simulink model "Drone2_simulink"  (R2024a)
settings: Solver=ode1be  StartTime=0.0  StopTime=1000  FixedStep=0.001  MaxStep=0.001  MinStep=0.00095  RelTol=1e-3
PreLoadFcn:
  | Drone_data;
model workspace: external: MATLAB File C:\Users\admin\OneDrive - Indian Institute of Technology Jodhpur\IIT JODHPUR\Research Work\Amphibious Drone\MATLAB_CODE\2025\New_Drone\Drone_1\Drone1_simulink_DataFile.m (data not in the file)
undefined symbols (not defined in the file): Environment, Newton, Raphson, Vehicle, X, Y, Z
libraries: sm_lib x1684, nesl_utility x63, slpidlib x25, eeGeneralControl x6, matrix_library x3, rllib x2, simulink x2, fl_lib x1, sharedutil x1, SignalEditorBlockLib x1
(part 3 of 17)

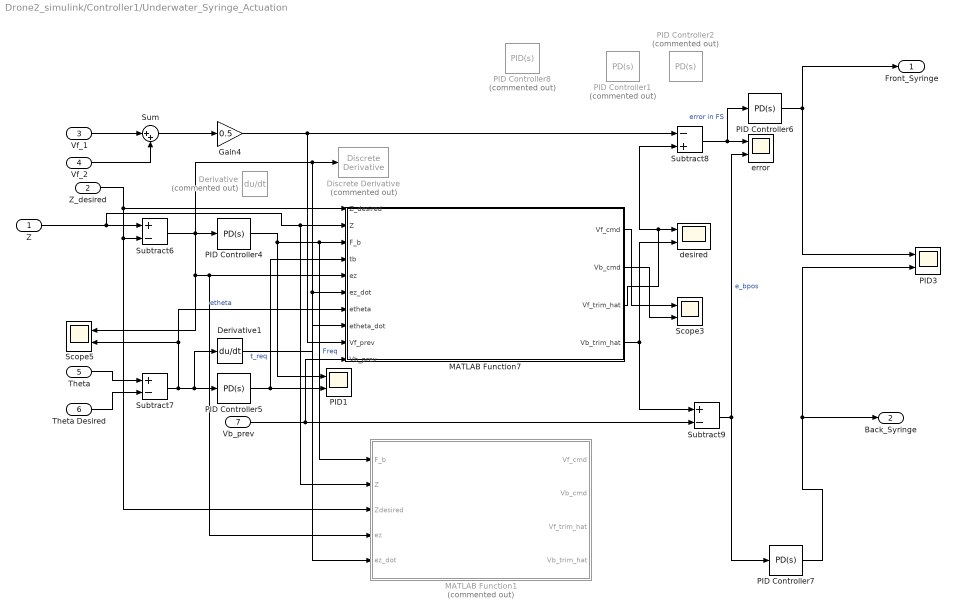
== system Drone2_simulink/Controller1/Underwater_Syringe_Actuation ==
  Z : Inport
  Z_desired : Inport  Port=2
  Vf_1 : Inport  Port=3
  Vf_2 : Inport  Port=4
  Theta : Inport  Port=5
  Theta Desired : Inport  Port=6
  Vb_prev : Inport  Port=7
  Derivative : Derivative  Commented=on
  Derivative1 : Derivative
  Discrete Derivative : simulink/Discrete/Discrete Derivative  Commented=on  gainval=1.0  ICPrevScaledInput=0.0  OutMin=[]  OutMax=[]  OutDataType=fixdt(1, 16)  OutScaling=2^-10  DoSatur=off
  Gain4 : Gain  Gain=0.5
  MATLAB Function1 : MATLAB Function  Commented=on  TreatAsAtomicUnit=on  mask{V_MIN=Vehicle.Syringe.Front.minpos, V_MAX=Vehicle.Syringe.Front.maxpos, V_DOT_MAX=0.012, HF=0.2, A=0, g=9.81, rho=1000, dt=0.001, Kp_pos=0.002, Kp_vel=0.002, Kr=0.005, EZDB=0.05, sigma=0.1, Ez_high=1, PLRate=0.0002, PKRate=0.05, ETDB=3}
      mask prompts: V_MIN "Min"; V_MAX "Max"; V_DOT_MAX "max rate"; HF "Half Length of drone"; A "Area of Syringe"; g "Gravity"; rho "Density"; dt "Sample Time"; Kp_pos "Learning Rate-Pose"; Kp_vel "Slow Learning Rate"; Kr "K_Rate"; EZDB "Error zone to reduce adaption"; sigma "Steady state error region"; Ez_high "mode switch region"; PLRate "Pitch Learning Rate"; PKRate "K_Rate"; ETDB "Error zone to reduce adaption"
  MATLAB Function7 : MATLAB Function  TreatAsAtomicUnit=on  mask{Min=Vehicle.Syringe.Front.minpos, Max=Vehicle.Syringe.Front.maxpos, HF=0.2, AS=0, G=9.81, RHO=1000, DT=0.001, DFRate=0.02, DMRate=0.002, DSRate=0.002, Dpanelty=0.005, EZDB=0.05, PLRate=0.0002, PKRate=0.05, ETDB=3}
      mask prompts: HF "Half Length of drone"; AS "Area of Syringe"; G "Gravity"; RHO "Density"; DT "Sample Time"; DFRate "Fast Learning rate with |e|>1"; DMRate "Medium Learning Rate"; DSRate "Slow Learning Rate"; Dpanelty "K_Rate"; EZDB "Error zone to reduce adaption"; PLRate "Pitch Learning Rate"; PKRate "K_Rate"; ETDB "Error zone to reduce adaption"
  PID Controller1 : slpidlib/PID Controller  Commented=on  Controller=PD  Form=Parallel  TimeDomain=Continuous-time  UseExternalTs=off  SampleTime=-1  IntegratorMethod=Forward Euler  FilterMethod=Forward Euler  ControllerParametersSource=internal  P=3500.0200194669353  I=843.52365195509  UseKiTs=on  D=26.9299392102605  UseExternalDerivativeSource=off  N=0.579906738639273  UseFilter=on  TunerSelectOption=Transfer Function Based (PID Tuner App)  InitialConditionSource=internal  InitialConditionForIntegrator=0  InitialConditionForFilter=0  DifferentiatorICPrevScaledInput=0  ExternalReset=none  TrackingMode=off  Kt=1  LimitOutput=on  SatLimitsSource=internal  UpperSaturationLimit=40  LowerSaturationLimit=0  LinearizeAsGain=on  AntiWindupMode=none  Kb=1  LimitIntegrator=off  UpperIntegratorSaturationLimit=inf  LowerIntegratorSaturationLimit=-inf  POutMin=[]  POutMax=[]  IOutMin=[]  IOutMax=[]  DOutMin=[]  DOutMax=[]  NOutMin=[]  NOutMax=[]  SumOutMin=[]  SumOutMax=[]  SaturationOutMin=[]  SaturationOutMax=[]  PParamMin=[]  PParamMax=[]  IParamMin=[]  IParamMax=[]  DParamMin=[]  DParamMax=[]  NParamMin=[]  NParamMax=[]  KbParamMin=[]  KbParamMax=[]  KtParamMin=[]  KtParamMax=[]  KbOutMin=[]  KbOutMax=[]  KtOutMin=[]  KtOutMax=[]  IntegratorOutMin=[]  IntegratorOutMax=[]  FilterOutMin=[]  FilterOutMax=[]  SumI1OutMin=[]  SumI1OutMax=[]  SumI2OutMin=[]  SumI2OutMax=[]  SumI3OutMin=[]  SumI3OutMax=[]  SumI4OutMin=[]  SumI4OutMax=[]  SumDOutMin=[]  SumDOutMax=[]  DifferentiatorOutMin=[]  DifferentiatorOutMax=[]  FilterDiffOutCoefMin=[]  FilterDiffOutCoefMax=[]  ReciprocalOutMin=[]  ReciprocalOutMax=[]  SumDenOutMin=[]  SumDenOutMax=[]  SumNumOutMin=[]  SumNumOutMax=[]  DivideOutMin=[]  DivideOutMax=[]  UdiffTsProdOutMin=[]  UdiffTsProdOutMax=[]  NTsProdOutMin=[]  NTsProdOutMax=[]  UintegralTsProdOutMin=[]  UintegralTsProdOutMax=[]  UngainTsProdOutMin=[]  UngainTsProdOutMax=[]  ClampingZeroOutDataTypeStr=Inherit: Inherit via back propagation  ClampingZeroOutMin=[]  ClampingZeroOutMax=[]  FilterDenConstantOutDataTypeStr=Inherit: Inherit via back propagation  FilterDenConstantOutMin=[]  FilterDenConstantOutMax=[]  PCopyOutDataTypeStr=Inherit: Inherit via back propagation  PCopyOutMin=[]  PCopyOutMax=[]  NCopyOutDataTypeStr=Inherit: Inherit via back propagation  NCopyOutMin=[]  NCopyOutMax=[]  IntegratorContinuousStateAttributes=''  IntegratorStateMustResolveToSignalObject=off  IntegratorRTWStateStorageClass=Auto  FilterContinuousStateAttributes=''  FilterStateMustResolveToSignalObject=off  FilterRTWStateStorageClass=Auto  ParallelPVariant=InternalParameters  IdealPVariant=Disabled  IVariant=Disabled  DVariant=InternalParameters  IntegratorVariant=Disabled  SatVariant=Enabled  AWVariant=Disabled  PCopyVariant=Disabled  TRVariant=Disabled  FdbkBlocksVariant=Forward  IdealPFdbkVariant=Disabled  SatFdbkVariant=Disabled  DerivativeFilterVariant=ContFilter  NVariant=InternalParameters  NCopyVariant=Disabled  FilterICVariant=InternalICsFilter  IntegratorICVariant=Disabled  ExternalResetVariant=Disabled  TRSumVariant=Passthrough  SumFdbkVariant=Disabled  SumVariant=Sum_PD  TsampFilterVariant=InternalTs  TsampNgainVariant=Passthrough  TsampIntegralVariant=Disabled_SignalSpec  ExternalSaturationOutDataTypeStr=Inherit: Same as second input  DerivativeSourceVariant=ErrorSignal
  PID Controller2 : slpidlib/PID Controller  Commented=on  Controller=PD  Form=Parallel  TimeDomain=Continuous-time  UseExternalTs=off  SampleTime=-1  IntegratorMethod=Forward Euler  FilterMethod=Forward Euler  ControllerParametersSource=internal  P=3744.13110896654  I=964.677966952311  UseKiTs=on  D=30  UseExternalDerivativeSource=off  N=0.58  UseFilter=on  TunerSelectOption=Transfer Function Based (PID Tuner App)  InitialConditionSource=internal  InitialConditionForIntegrator=0  InitialConditionForFilter=0  DifferentiatorICPrevScaledInput=0  ExternalReset=none  TrackingMode=off  Kt=1  LimitOutput=on  SatLimitsSource=internal  UpperSaturationLimit=40  LowerSaturationLimit=0  LinearizeAsGain=on  AntiWindupMode=none  Kb=1  LimitIntegrator=off  UpperIntegratorSaturationLimit=inf  LowerIntegratorSaturationLimit=-inf  POutMin=[]  POutMax=[]  IOutMin=[]  IOutMax=[]  DOutMin=[]  DOutMax=[]  NOutMin=[]  NOutMax=[]  SumOutMin=[]  SumOutMax=[]  SaturationOutMin=[]  SaturationOutMax=[]  PParamMin=[]  PParamMax=[]  IParamMin=[]  IParamMax=[]  DParamMin=[]  DParamMax=[]  NParamMin=[]  NParamMax=[]  KbParamMin=[]  KbParamMax=[]  KtParamMin=[]  KtParamMax=[]  KbOutMin=[]  KbOutMax=[]  KtOutMin=[]  KtOutMax=[]  IntegratorOutMin=[]  IntegratorOutMax=[]  FilterOutMin=[]  FilterOutMax=[]  SumI1OutMin=[]  SumI1OutMax=[]  SumI2OutMin=[]  SumI2OutMax=[]  SumI3OutMin=[]  SumI3OutMax=[]  SumI4OutMin=[]  SumI4OutMax=[]  SumDOutMin=[]  SumDOutMax=[]  DifferentiatorOutMin=[]  DifferentiatorOutMax=[]  FilterDiffOutCoefMin=[]  FilterDiffOutCoefMax=[]  ReciprocalOutMin=[]  ReciprocalOutMax=[]  SumDenOutMin=[]  SumDenOutMax=[]  SumNumOutMin=[]  SumNumOutMax=[]  DivideOutMin=[]  DivideOutMax=[]  UdiffTsProdOutMin=[]  UdiffTsProdOutMax=[]  NTsProdOutMin=[]  NTsProdOutMax=[]  UintegralTsProdOutMin=[]  UintegralTsProdOutMax=[]  UngainTsProdOutMin=[]  UngainTsProdOutMax=[]  ClampingZeroOutDataTypeStr=Inherit: Inherit via back propagation  ClampingZeroOutMin=[]  ClampingZeroOutMax=[]  FilterDenConstantOutDataTypeStr=Inherit: Inherit via back propagation  FilterDenConstantOutMin=[]  FilterDenConstantOutMax=[]  PCopyOutDataTypeStr=Inherit: Inherit via back propagation  PCopyOutMin=[]  PCopyOutMax=[]  NCopyOutDataTypeStr=Inherit: Inherit via back propagation  NCopyOutMin=[]  NCopyOutMax=[]  IntegratorContinuousStateAttributes=''  IntegratorStateMustResolveToSignalObject=off  IntegratorRTWStateStorageClass=Auto  FilterContinuousStateAttributes=''  FilterStateMustResolveToSignalObject=off  FilterRTWStateStorageClass=Auto  ParallelPVariant=InternalParameters  IdealPVariant=Disabled  IVariant=Disabled  DVariant=InternalParameters  IntegratorVariant=Disabled  SatVariant=Enabled  AWVariant=Disabled  PCopyVariant=Disabled  TRVariant=Disabled  FdbkBlocksVariant=Forward  IdealPFdbkVariant=Disabled  SatFdbkVariant=Disabled  DerivativeFilterVariant=ContFilter  NVariant=InternalParameters  NCopyVariant=Disabled  FilterICVariant=InternalICsFilter  IntegratorICVariant=Disabled  ExternalResetVariant=Disabled  TRSumVariant=Passthrough  SumFdbkVariant=Disabled  SumVariant=Sum_PD  TsampFilterVariant=InternalTs  TsampNgainVariant=Passthrough  TsampIntegralVariant=Disabled_SignalSpec  ExternalSaturationOutDataTypeStr=Inherit: Same as second input  DerivativeSourceVariant=ErrorSignal
  PID Controller4 : slpidlib/PID Controller  Controller=PD  Form=Parallel  TimeDomain=Continuous-time  UseExternalTs=off  SampleTime=-1  IntegratorMethod=Forward Euler  FilterMethod=Forward Euler  ControllerParametersSource=internal  P=8  I=0  UseKiTs=on  D=0.5  UseExternalDerivativeSource=off  N=20  UseFilter=on  TunerSelectOption=Transfer Function Based (PID Tuner App)  InitialConditionSource=internal  InitialConditionForIntegrator=0  InitialConditionForFilter=0  DifferentiatorICPrevScaledInput=0  ExternalReset=none  TrackingMode=off  Kt=1  LimitOutput=off  SatLimitsSource=internal  UpperSaturationLimit=Vehicle.Syringe.Thrustlim  LowerSaturationLimit=-Vehicle.Syringe.Thrustlim  LinearizeAsGain=on  AntiWindupMode=none  Kb=1  LimitIntegrator=off  UpperIntegratorSaturationLimit=inf  LowerIntegratorSaturationLimit=-inf  POutMin=[]  POutMax=[]  IOutMin=[]  IOutMax=[]  DOutMin=[]  DOutMax=[]  NOutMin=[]  NOutMax=[]  SumOutMin=[]  SumOutMax=[]  SaturationOutMin=[]  SaturationOutMax=[]  PParamMin=[]  PParamMax=[]  IParamMin=[]  IParamMax=[]  DParamMin=[]  DParamMax=[]  NParamMin=[]  NParamMax=[]  KbParamMin=[]  KbParamMax=[]  KtParamMin=[]  KtParamMax=[]  KbOutMin=[]  KbOutMax=[]  KtOutMin=[]  KtOutMax=[]  IntegratorOutMin=[]  IntegratorOutMax=[]  FilterOutMin=[]  FilterOutMax=[]  SumI1OutMin=[]  SumI1OutMax=[]  SumI2OutMin=[]  SumI2OutMax=[]  SumI3OutMin=[]  SumI3OutMax=[]  SumI4OutMin=[]  SumI4OutMax=[]  SumDOutMin=[]  SumDOutMax=[]  DifferentiatorOutMin=[]  DifferentiatorOutMax=[]  FilterDiffOutCoefMin=[]  FilterDiffOutCoefMax=[]  ReciprocalOutMin=[]  ReciprocalOutMax=[]  SumDenOutMin=[]  SumDenOutMax=[]  SumNumOutMin=[]  SumNumOutMax=[]  DivideOutMin=[]  DivideOutMax=[]  UdiffTsProdOutMin=[]  UdiffTsProdOutMax=[]  NTsProdOutMin=[]  NTsProdOutMax=[]  UintegralTsProdOutMin=[]  UintegralTsProdOutMax=[]  UngainTsProdOutMin=[]  UngainTsProdOutMax=[]  ClampingZeroOutDataTypeStr=Inherit: Inherit via back propagation  ClampingZeroOutMin=[]  ClampingZeroOutMax=[]  FilterDenConstantOutDataTypeStr=Inherit: Inherit via back propagation  FilterDenConstantOutMin=[]  FilterDenConstantOutMax=[]  PCopyOutDataTypeStr=Inherit: Inherit via back propagation  PCopyOutMin=[]  PCopyOutMax=[]  NCopyOutDataTypeStr=Inherit: Inherit via back propagation  NCopyOutMin=[]  NCopyOutMax=[]  IntegratorContinuousStateAttributes=''  IntegratorStateMustResolveToSignalObject=off  IntegratorRTWStateStorageClass=Auto  FilterContinuousStateAttributes=''  FilterStateMustResolveToSignalObject=off  FilterRTWStateStorageClass=Auto  ParallelPVariant=InternalParameters  IdealPVariant=Disabled  IVariant=Disabled  DVariant=InternalParameters  IntegratorVariant=Disabled  SatVariant=Disabled  AWVariant=Disabled  PCopyVariant=Disabled  TRVariant=Disabled  FdbkBlocksVariant=Forward  IdealPFdbkVariant=Disabled  SatFdbkVariant=Disabled  DerivativeFilterVariant=ContFilter  NVariant=InternalParameters  NCopyVariant=Disabled  FilterICVariant=InternalICsFilter  IntegratorICVariant=Disabled  ExternalResetVariant=Disabled  TRSumVariant=Passthrough  SumFdbkVariant=Disabled  SumVariant=Sum_PD  TsampFilterVariant=InternalTs  TsampNgainVariant=Passthrough  TsampIntegralVariant=Disabled_SignalSpec  ExternalSaturationOutDataTypeStr=Inherit: Same as second input  DerivativeSourceVariant=ErrorSignal
  PID Controller5 : slpidlib/PID Controller  Controller=PD  Form=Parallel  TimeDomain=Continuous-time  UseExternalTs=off  SampleTime=-1  IntegratorMethod=Forward Euler  FilterMethod=Forward Euler  ControllerParametersSource=internal  P=4  I=0  UseKiTs=on  D=0.5  UseExternalDerivativeSource=off  N=100  UseFilter=on  TunerSelectOption=Transfer Function Based (PID Tuner App)  InitialConditionSource=internal  InitialConditionForIntegrator=0  InitialConditionForFilter=0  DifferentiatorICPrevScaledInput=0  ExternalReset=none  TrackingMode=off  Kt=1  LimitOutput=off  SatLimitsSource=internal  UpperSaturationLimit=Vehicle.Syringe.Thrustlim  LowerSaturationLimit=-Vehicle.Syringe.Thrustlim  LinearizeAsGain=on  AntiWindupMode=none  Kb=1  LimitIntegrator=off  UpperIntegratorSaturationLimit=inf  LowerIntegratorSaturationLimit=-inf  POutMin=[]  POutMax=[]  IOutMin=[]  IOutMax=[]  DOutMin=[]  DOutMax=[]  NOutMin=[]  NOutMax=[]  SumOutMin=[]  SumOutMax=[]  SaturationOutMin=[]  SaturationOutMax=[]  PParamMin=[]  PParamMax=[]  IParamMin=[]  IParamMax=[]  DParamMin=[]  DParamMax=[]  NParamMin=[]  NParamMax=[]  KbParamMin=[]  KbParamMax=[]  KtParamMin=[]  KtParamMax=[]  KbOutMin=[]  KbOutMax=[]  KtOutMin=[]  KtOutMax=[]  IntegratorOutMin=[]  IntegratorOutMax=[]  FilterOutMin=[]  FilterOutMax=[]  SumI1OutMin=[]  SumI1OutMax=[]  SumI2OutMin=[]  SumI2OutMax=[]  SumI3OutMin=[]  SumI3OutMax=[]  SumI4OutMin=[]  SumI4OutMax=[]  SumDOutMin=[]  SumDOutMax=[]  DifferentiatorOutMin=[]  DifferentiatorOutMax=[]  FilterDiffOutCoefMin=[]  FilterDiffOutCoefMax=[]  ReciprocalOutMin=[]  ReciprocalOutMax=[]  SumDenOutMin=[]  SumDenOutMax=[]  SumNumOutMin=[]  SumNumOutMax=[]  DivideOutMin=[]  DivideOutMax=[]  UdiffTsProdOutMin=[]  UdiffTsProdOutMax=[]  NTsProdOutMin=[]  NTsProdOutMax=[]  UintegralTsProdOutMin=[]  UintegralTsProdOutMax=[]  UngainTsProdOutMin=[]  UngainTsProdOutMax=[]  ClampingZeroOutDataTypeStr=Inherit: Inherit via back propagation  ClampingZeroOutMin=[]  ClampingZeroOutMax=[]  FilterDenConstantOutDataTypeStr=Inherit: Inherit via back propagation  FilterDenConstantOutMin=[]  FilterDenConstantOutMax=[]  PCopyOutDataTypeStr=Inherit: Inherit via back propagation  PCopyOutMin=[]  PCopyOutMax=[]  NCopyOutDataTypeStr=Inherit: Inherit via back propagation  NCopyOutMin=[]  NCopyOutMax=[]  IntegratorContinuousStateAttributes=''  IntegratorStateMustResolveToSignalObject=off  IntegratorRTWStateStorageClass=Auto  FilterContinuousStateAttributes=''  FilterStateMustResolveToSignalObject=off  FilterRTWStateStorageClass=Auto  ParallelPVariant=InternalParameters  IdealPVariant=Disabled  IVariant=Disabled  DVariant=InternalParameters  IntegratorVariant=Disabled  SatVariant=Disabled  AWVariant=Disabled  PCopyVariant=Disabled  TRVariant=Disabled  FdbkBlocksVariant=Forward  IdealPFdbkVariant=Disabled  SatFdbkVariant=Disabled  DerivativeFilterVariant=ContFilter  NVariant=InternalParameters  NCopyVariant=Disabled  FilterICVariant=InternalICsFilter  IntegratorICVariant=Disabled  ExternalResetVariant=Disabled  TRSumVariant=Passthrough  SumFdbkVariant=Disabled  SumVariant=Sum_PD  TsampFilterVariant=InternalTs  TsampNgainVariant=Passthrough  TsampIntegralVariant=Disabled_SignalSpec  ExternalSaturationOutDataTypeStr=Inherit: Same as second input  DerivativeSourceVariant=ErrorSignal
  PID Controller6 : slpidlib/PID Controller  Controller=PD  Form=Parallel  TimeDomain=Continuous-time  UseExternalTs=off  SampleTime=-1  IntegratorMethod=Forward Euler  FilterMethod=Forward Euler  ControllerParametersSource=internal  P=3500  I=843.52365195509  UseKiTs=on  D=30  UseExternalDerivativeSource=off  N=1  UseFilter=on  TunerSelectOption=Transfer Function Based (PID Tuner App)  InitialConditionSource=internal  InitialConditionForIntegrator=0  InitialConditionForFilter=0  DifferentiatorICPrevScaledInput=0  ExternalReset=none  TrackingMode=off  Kt=1  LimitOutput=on  SatLimitsSource=internal  UpperSaturationLimit=40  LowerSaturationLimit=0  LinearizeAsGain=on  AntiWindupMode=none  Kb=1  LimitIntegrator=off  UpperIntegratorSaturationLimit=inf  LowerIntegratorSaturationLimit=-inf  POutMin=[]  POutMax=[]  IOutMin=[]  IOutMax=[]  DOutMin=[]  DOutMax=[]  NOutMin=[]  NOutMax=[]  SumOutMin=[]  SumOutMax=[]  SaturationOutMin=[]  SaturationOutMax=[]  PParamMin=[]  PParamMax=[]  IParamMin=[]  IParamMax=[]  DParamMin=[]  DParamMax=[]  NParamMin=[]  NParamMax=[]  KbParamMin=[]  KbParamMax=[]  KtParamMin=[]  KtParamMax=[]  KbOutMin=[]  KbOutMax=[]  KtOutMin=[]  KtOutMax=[]  IntegratorOutMin=[]  IntegratorOutMax=[]  FilterOutMin=[]  FilterOutMax=[]  SumI1OutMin=[]  SumI1OutMax=[]  SumI2OutMin=[]  SumI2OutMax=[]  SumI3OutMin=[]  SumI3OutMax=[]  SumI4OutMin=[]  SumI4OutMax=[]  SumDOutMin=[]  SumDOutMax=[]  DifferentiatorOutMin=[]  DifferentiatorOutMax=[]  FilterDiffOutCoefMin=[]  FilterDiffOutCoefMax=[]  ReciprocalOutMin=[]  ReciprocalOutMax=[]  SumDenOutMin=[]  SumDenOutMax=[]  SumNumOutMin=[]  SumNumOutMax=[]  DivideOutMin=[]  DivideOutMax=[]  UdiffTsProdOutMin=[]  UdiffTsProdOutMax=[]  NTsProdOutMin=[]  NTsProdOutMax=[]  UintegralTsProdOutMin=[]  UintegralTsProdOutMax=[]  UngainTsProdOutMin=[]  UngainTsProdOutMax=[]  ClampingZeroOutDataTypeStr=Inherit: Inherit via back propagation  ClampingZeroOutMin=[]  ClampingZeroOutMax=[]  FilterDenConstantOutDataTypeStr=Inherit: Inherit via back propagation  FilterDenConstantOutMin=[]  FilterDenConstantOutMax=[]  PCopyOutDataTypeStr=Inherit: Inherit via back propagation  PCopyOutMin=[]  PCopyOutMax=[]  NCopyOutDataTypeStr=Inherit: Inherit via back propagation  NCopyOutMin=[]  NCopyOutMax=[]  IntegratorContinuousStateAttributes=''  IntegratorStateMustResolveToSignalObject=off  IntegratorRTWStateStorageClass=Auto  FilterContinuousStateAttributes=''  FilterStateMustResolveToSignalObject=off  FilterRTWStateStorageClass=Auto  ParallelPVariant=InternalParameters  IdealPVariant=Disabled  IVariant=Disabled  DVariant=InternalParameters  IntegratorVariant=Disabled  SatVariant=Enabled  AWVariant=Disabled  PCopyVariant=Disabled  TRVariant=Disabled  FdbkBlocksVariant=Forward  IdealPFdbkVariant=Disabled  SatFdbkVariant=Disabled  DerivativeFilterVariant=ContFilter  NVariant=InternalParameters  NCopyVariant=Disabled  FilterICVariant=InternalICsFilter  IntegratorICVariant=Disabled  ExternalResetVariant=Disabled  TRSumVariant=Passthrough  SumFdbkVariant=Disabled  SumVariant=Sum_PD  TsampFilterVariant=InternalTs  TsampNgainVariant=Passthrough  TsampIntegralVariant=Disabled_SignalSpec  ExternalSaturationOutDataTypeStr=Inherit: Same as second input  DerivativeSourceVariant=ErrorSignal
  PID Controller7 : slpidlib/PID Controller  Controller=PD  Form=Parallel  TimeDomain=Continuous-time  UseExternalTs=off  SampleTime=-1  IntegratorMethod=Forward Euler  FilterMethod=Forward Euler  ControllerParametersSource=internal  P=3750  I=964.677966952311  UseKiTs=on  D=30  UseExternalDerivativeSource=off  N=1  UseFilter=on  TunerSelectOption=Transfer Function Based (PID Tuner App)  InitialConditionSource=internal  InitialConditionForIntegrator=0  InitialConditionForFilter=0  DifferentiatorICPrevScaledInput=0  ExternalReset=none  TrackingMode=off  Kt=1  LimitOutput=on  SatLimitsSource=internal  UpperSaturationLimit=40  LowerSaturationLimit=0  LinearizeAsGain=on  AntiWindupMode=none  Kb=1  LimitIntegrator=off  UpperIntegratorSaturationLimit=inf  LowerIntegratorSaturationLimit=-inf  POutMin=[]  POutMax=[]  IOutMin=[]  IOutMax=[]  DOutMin=[]  DOutMax=[]  NOutMin=[]  NOutMax=[]  SumOutMin=[]  SumOutMax=[]  SaturationOutMin=[]  SaturationOutMax=[]  PParamMin=[]  PParamMax=[]  IParamMin=[]  IParamMax=[]  DParamMin=[]  DParamMax=[]  NParamMin=[]  NParamMax=[]  KbParamMin=[]  KbParamMax=[]  KtParamMin=[]  KtParamMax=[]  KbOutMin=[]  KbOutMax=[]  KtOutMin=[]  KtOutMax=[]  IntegratorOutMin=[]  IntegratorOutMax=[]  FilterOutMin=[]  FilterOutMax=[]  SumI1OutMin=[]  SumI1OutMax=[]  SumI2OutMin=[]  SumI2OutMax=[]  SumI3OutMin=[]  SumI3OutMax=[]  SumI4OutMin=[]  SumI4OutMax=[]  SumDOutMin=[]  SumDOutMax=[]  DifferentiatorOutMin=[]  DifferentiatorOutMax=[]  FilterDiffOutCoefMin=[]  FilterDiffOutCoefMax=[]  ReciprocalOutMin=[]  ReciprocalOutMax=[]  SumDenOutMin=[]  SumDenOutMax=[]  SumNumOutMin=[]  SumNumOutMax=[]  DivideOutMin=[]  DivideOutMax=[]  UdiffTsProdOutMin=[]  UdiffTsProdOutMax=[]  NTsProdOutMin=[]  NTsProdOutMax=[]  UintegralTsProdOutMin=[]  UintegralTsProdOutMax=[]  UngainTsProdOutMin=[]  UngainTsProdOutMax=[]  ClampingZeroOutDataTypeStr=Inherit: Inherit via back propagation  ClampingZeroOutMin=[]  ClampingZeroOutMax=[]  FilterDenConstantOutDataTypeStr=Inherit: Inherit via back propagation  FilterDenConstantOutMin=[]  FilterDenConstantOutMax=[]  PCopyOutDataTypeStr=Inherit: Inherit via back propagation  PCopyOutMin=[]  PCopyOutMax=[]  NCopyOutDataTypeStr=Inherit: Inherit via back propagation  NCopyOutMin=[]  NCopyOutMax=[]  IntegratorContinuousStateAttributes=''  IntegratorStateMustResolveToSignalObject=off  IntegratorRTWStateStorageClass=Auto  FilterContinuousStateAttributes=''  FilterStateMustResolveToSignalObject=off  FilterRTWStateStorageClass=Auto  ParallelPVariant=InternalParameters  IdealPVariant=Disabled  IVariant=Disabled  DVariant=InternalParameters  IntegratorVariant=Disabled  SatVariant=Enabled  AWVariant=Disabled  PCopyVariant=Disabled  TRVariant=Disabled  FdbkBlocksVariant=Forward  IdealPFdbkVariant=Disabled  SatFdbkVariant=Disabled  DerivativeFilterVariant=ContFilter  NVariant=InternalParameters  NCopyVariant=Disabled  FilterICVariant=InternalICsFilter  IntegratorICVariant=Disabled  ExternalResetVariant=Disabled  TRSumVariant=Passthrough  SumFdbkVariant=Disabled  SumVariant=Sum_PD  TsampFilterVariant=InternalTs  TsampNgainVariant=Passthrough  TsampIntegralVariant=Disabled_SignalSpec  ExternalSaturationOutDataTypeStr=Inherit: Same as second input  DerivativeSourceVariant=ErrorSignal
  PID Controller8 : slpidlib/PID Controller  Commented=on  Controller=PID  Form=Parallel  TimeDomain=Continuous-time  UseExternalTs=off  SampleTime=-1  IntegratorMethod=Forward Euler  FilterMethod=Forward Euler  ControllerParametersSource=internal  P=44.1440048797783  I=843.52365195509  UseKiTs=on  D=0  UseExternalDerivativeSource=off  N=100  UseFilter=on  TunerSelectOption=Transfer Function Based (PID Tuner App)  InitialConditionSource=internal  InitialConditionForIntegrator=0  InitialConditionForFilter=0  DifferentiatorICPrevScaledInput=0  ExternalReset=none  TrackingMode=off  Kt=1  LimitOutput=on  SatLimitsSource=internal  UpperSaturationLimit=40  LowerSaturationLimit=0  LinearizeAsGain=on  AntiWindupMode=none  Kb=1  LimitIntegrator=off  UpperIntegratorSaturationLimit=inf  LowerIntegratorSaturationLimit=-inf  POutMin=[]  POutMax=[]  IOutMin=[]  IOutMax=[]  DOutMin=[]  DOutMax=[]  NOutMin=[]  NOutMax=[]  SumOutMin=[]  SumOutMax=[]  SaturationOutMin=[]  SaturationOutMax=[]  PParamMin=[]  PParamMax=[]  IParamMin=[]  IParamMax=[]  DParamMin=[]  DParamMax=[]  NParamMin=[]  NParamMax=[]  KbParamMin=[]  KbParamMax=[]  KtParamMin=[]  KtParamMax=[]  KbOutMin=[]  KbOutMax=[]  KtOutMin=[]  KtOutMax=[]  IntegratorOutMin=[]  IntegratorOutMax=[]  FilterOutMin=[]  FilterOutMax=[]  SumI1OutMin=[]  SumI1OutMax=[]  SumI2OutMin=[]  SumI2OutMax=[]  SumI3OutMin=[]  SumI3OutMax=[]  SumI4OutMin=[]  SumI4OutMax=[]  SumDOutMin=[]  SumDOutMax=[]  DifferentiatorOutMin=[]  DifferentiatorOutMax=[]  FilterDiffOutCoefMin=[]  FilterDiffOutCoefMax=[]  ReciprocalOutMin=[]  ReciprocalOutMax=[]  SumDenOutMin=[]  SumDenOutMax=[]  SumNumOutMin=[]  SumNumOutMax=[]  DivideOutMin=[]  DivideOutMax=[]  UdiffTsProdOutMin=[]  UdiffTsProdOutMax=[]  NTsProdOutMin=[]  NTsProdOutMax=[]  UintegralTsProdOutMin=[]  UintegralTsProdOutMax=[]  UngainTsProdOutMin=[]  UngainTsProdOutMax=[]  ClampingZeroOutDataTypeStr=Inherit: Inherit via back propagation  ClampingZeroOutMin=[]  ClampingZeroOutMax=[]  FilterDenConstantOutDataTypeStr=Inherit: Inherit via back propagation  FilterDenConstantOutMin=[]  FilterDenConstantOutMax=[]  PCopyOutDataTypeStr=Inherit: Inherit via back propagation  PCopyOutMin=[]  PCopyOutMax=[]  NCopyOutDataTypeStr=Inherit: Inherit via back propagation  NCopyOutMin=[]  NCopyOutMax=[]  IntegratorContinuousStateAttributes=''  IntegratorStateMustResolveToSignalObject=off  IntegratorRTWStateStorageClass=Auto  FilterContinuousStateAttributes=''  FilterStateMustResolveToSignalObject=off  FilterRTWStateStorageClass=Auto  ParallelPVariant=InternalParameters  IdealPVariant=Disabled  IVariant=InternalParameters  DVariant=InternalParameters  IntegratorVariant=Continuous  SatVariant=Enabled  AWVariant=Passthrough  PCopyVariant=Disabled  TRVariant=Disabled  FdbkBlocksVariant=Forward  IdealPFdbkVariant=Disabled  SatFdbkVariant=Disabled  DerivativeFilterVariant=ContFilter  NVariant=InternalParameters  NCopyVariant=Disabled  FilterICVariant=InternalICsFilter  IntegratorICVariant=InternalICs  ExternalResetVariant=Disabled  TRSumVariant=Passthrough  SumFdbkVariant=Disabled  SumVariant=Sum_PID  TsampFilterVariant=InternalTs  TsampNgainVariant=Passthrough  TsampIntegralVariant=Disabled_SignalSpec  ExternalSaturationOutDataTypeStr=Inherit: Same as second input  DerivativeSourceVariant=ErrorSignal
  PID1 : Scope  NumInputPorts=2
  PID3 : Scope  NumInputPorts=2
  Scope3 : Scope  NumInputPorts=2
  Scope5 : Scope  NumInputPorts=2
  Subtract6 : Sum  Inputs=+-
  Subtract7 : Sum  Inputs=+-
  Subtract8 : Sum  Inputs=-+
  Subtract9 : Sum  Inputs=+-
  Sum : Sum  Inputs=|++
  desired : Scope  NumInputPorts=2
  error : Scope  NumInputPorts=2
  Front_Syringe : Outport
  Back_Syringe : Outport  Port=2
  wires:
  Subtract6/1 -> PID Controller4/1, MATLAB Function7/5(ez), MATLAB Function1/4(ez), Scope5/1, MATLAB Function7/6(ez_dot), MATLAB Function1/5(ez_dot), Discrete Derivative/1
  Z_desired/1 -> Subtract6/2, MATLAB Function1/3(Zdesired), MATLAB Function7/1(Z_desired)
  PID Controller7/1 -> Back_Syringe/1, PID3/2
  PID Controller6/1 -> Front_Syringe/1, PID3/1
  MATLAB Function7/4(Vb_trim_hat) -> desired/2, Subtract9/1
  MATLAB Function7/3(Vf_trim_hat) -> desired/1, Subtract8/2
  Vb_prev/1 -> MATLAB Function7/10(Vb_prev), Subtract9/2
  PID Controller5/1 -> PID1/2, MATLAB Function7/4(tb)  "t_req"
  MATLAB Function7/1(Vf_cmd) -> Scope3/1
  Derivative1/1 -> MATLAB Function7/8(etheta_dot)
  PID Controller4/1 -> PID1/1, MATLAB Function7/3(F_b), MATLAB Function1/1(F_b)  "Freq"
  Gain4/1 -> MATLAB Function7/9(Vf_prev), Subtract8/1
  Subtract7/1 -> PID Controller5/1, Derivative1/1, MATLAB Function7/7(etheta), Scope5/2  "etheta"
  Theta Desired/1 -> Subtract7/2
  Theta/1 -> Subtract7/1
  Sum/1 -> Gain4/1
  Z/1 -> Subtract6/1, MATLAB Function7/2(Z), MATLAB Function1/2(Z)
  Subtract8/1 -> PID Controller6/1, error/1  "error in FS"
  MATLAB Function7/2(Vb_cmd) -> Scope3/2
  Vf_2/1 -> Sum/2
  Vf_1/1 -> Sum/1
  Subtract9/1 -> PID Controller7/1, error/2  "e_bpos"

== system Drone2_simulink/Drive Controls/Thrust Controls ==
  Bus Element In : Inport  PortName=Reference  Element=Speed
  Bus Element In2 : Inport  PortName=Reference  Element=Depth
  Bus Element In7 : Inport  PortName=Reference  Element=Heading
  Bus Element In1 : Inport  Port=2  PortName=VehicleFDBK  Element=COM.Body.Vb.u
  Bus Element In8 : Inport  Port=2  PortName=VehicleFDBK  Element=COM.Body.Vb.v
  Bus Element In5 : Inport  Port=2  PortName=VehicleFDBK  Element=COM.Body.wb
  Bus Element In6 : Inport  Port=2  PortName=VehicleFDBK  Element=COM.Derived.Euler
  Bus Element In3 : Inport  Port=2  PortName=VehicleFDBK  Element=COM.Derived.Euler.theta
  Bus Element In4 : Inport  Port=2  PortName=VehicleFDBK  Element=COM.World.Xe.Z
  Depth and Pitch Control : Subsystem
  Heading and Yaw Control : Subsystem
  Longitudinal Speed (Surge) Control : Subsystem
  PPf : Outport
  SPf : Outport  Port=2
  BVTf : Outport  Port=3
  SVTf : Outport  Port=4
  BHTf : Outport  Port=5
  SHTf : Outport  Port=6
  wires:
  Longitudinal Speed (Surge) Control/1(PPfcmd) -> Depth and Pitch Control/1(PPf), PPf/1
  Bus Element In/1 -> Longitudinal Speed (Surge) Control/1(uRef)
  Bus Element In1/1 -> Longitudinal Speed (Surge) Control/2(u)
  Longitudinal Speed (Surge) Control/2(SPfcmd) -> Depth and Pitch Control/2(SPf), SPf/1
  Depth and Pitch Control/2(SVTfcmd) -> SVTf/1
  Depth and Pitch Control/1(BVTfcmd) -> BVTf/1
  Heading and Yaw Control/1(BHTfcmd) -> BHTf/1
  Heading and Yaw Control/2(SHTfcmd) -> SHTf/1
  Bus Element In2/1 -> Depth and Pitch Control/3(ZRef)
  Bus Element In3/1 -> Depth and Pitch Control/5(theta)
  Bus Element In4/1 -> Depth and Pitch Control/4(Z)
  Bus Element In5/1 -> Heading and Yaw Control/3(pqr)
  Bus Element In6/1 -> Heading and Yaw Control/4(phithetapsi)
  Bus Element In7/1 -> Heading and Yaw Control/2(psiRef)
  Bus Element In8/1 -> Heading and Yaw Control/1(v)

== system Drone2_simulink/Drive Controls/Torque Controls ==
  Tbht (N*m) : Constant  Value=0
  Tbvt (N*m) : Constant  Value=0
  Tpp (N*m) : Constant  Value=0
  Tsht (N*m) : Constant  Value=0
  Tsp (N*m) : Constant  Value=0
  Tsvt (N*m) : Constant  Value=0
  BHTt : Outport
  BVTt : Outport  Port=2
  PPt : Outport  Port=3
  SPt : Outport  Port=4
  SHTt : Outport  Port=5
  SVTt : Outport  Port=6
  wires:
  Tbht (N*m)/1 -> BHTt/1
  Tsvt (N*m)/1 -> SVTt/1
  Tpp (N*m)/1 -> PPt/1
  Tsp (N*m)/1 -> SPt/1
  Tbvt (N*m)/1 -> BVTt/1
  Tsht (N*m)/1 -> SHTt/1

== system Drone2_simulink/Hydrostatic & Hydrodynamic Effects/Added Mass Forces ==
  Vb : Inport
  wb : Inport  Port=2
  Abb : Inport  Port=3
  dwbdt : Inport  Port=4
  Added Mass : Subsystem
  Added Mass Matrix : Constant  Value=Vehicle.AddedMassMatrix
  Coriolis : Subsystem
  Scope : Scope  NumInputPorts=2
  Scope1 : Scope  NumInputPorts=2
  Bus Element Out : Outport  PortName=AddedMass  Element=AMForcesXYZ
  Bus Element Out1 : Outport  PortName=AddedMass  Element=AMMomentsXYZ
  Bus Element Out2 : Outport  PortName=AddedMass  Element=CForcesXYZ
  Bus Element Out3 : Outport  PortName=AddedMass  Element=CMomentsXYZ
  wires:
  Added Mass Matrix/1 -> Added Mass/1(Ma), Coriolis/3(Ma)
  Abb/1 -> Added Mass/2(Abb)
  dwbdt/1 -> Added Mass/3(dwbdt)
  Added Mass/1(Fxyz) -> Scope/2, Bus Element Out/1
  Added Mass/2(Mxyz) -> Scope1/2, Bus Element Out1/1
  Vb/1 -> Coriolis/1(Vb)
  wb/1 -> Coriolis/2(wb)
  Coriolis/2(Mxyz) -> Scope1/1, Bus Element Out3/1
  Coriolis/1(Fxyz) -> Scope/1, Bus Element Out2/1

== system Drone2_simulink/Hydrostatic & Hydrodynamic Effects/Buoyancy Force ==
  Z : Inport
  Constant : Constant  Value=-Vehicle.Dist.CGtoTop
  Constant1 : Constant  Value=Vehicle.Dist.CGtoBottom
  Constant2 : Constant
  Constant3 : Constant  Value=0
  Constant4 : Constant  Value=Vehicle.MaxBuoyancyForce
  MATLAB Function : MATLAB Function  TreatAsAtomicUnit=on
  Product : Product
  Saturation : Saturate  UpperLimit=Vehicle.Dist.CGtoBottom  LowerLimit=-Vehicle.Dist.CGtoTop
  Scope : Scope  NumInputPorts=2
  Buoyancy force : Outport
  wires:
  Constant/1 -> MATLAB Function/2(a)
  Constant3/1 -> MATLAB Function/6(reverse), MATLAB Function/5(y_b)
  Constant4/1 -> Product/2
  Z/1 -> Saturation/1
  Constant1/1 -> MATLAB Function/3(b)
  Constant2/1 -> MATLAB Function/4(y_a)
  MATLAB Function/1(Factor) -> Product/1, Scope/1
  Product/1 -> Scope/2, Buoyancy force/1
  Saturation/1 -> MATLAB Function/1(Z)

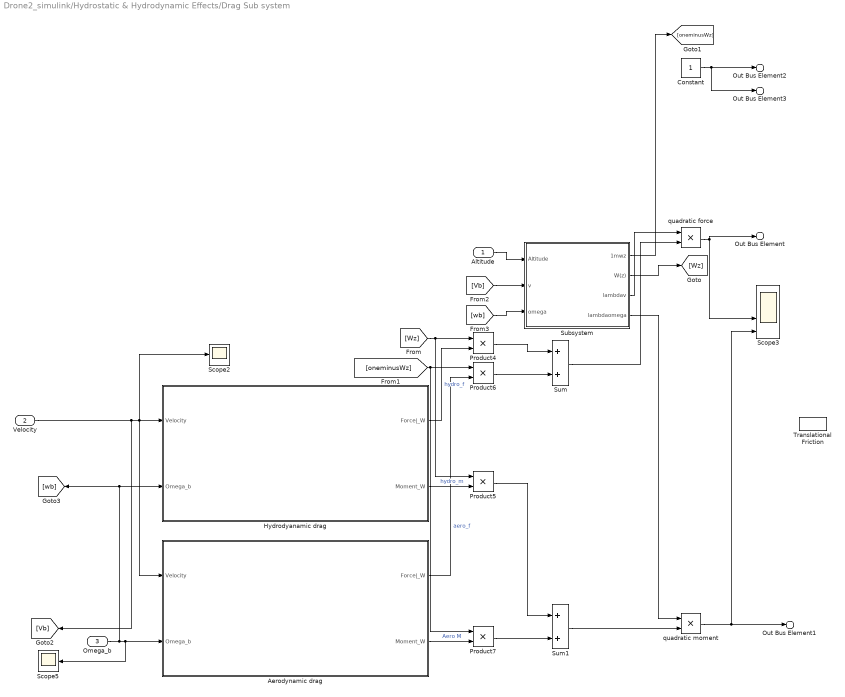
== system Drone2_simulink/Hydrostatic & Hydrodynamic Effects/Drag Sub system ==
  Altitude : Inport
  Velocity : Inport  Port=2
  Omega_b : Inport  Port=3
  Aerodynamic drag : Subsystem
  Constant : Constant
  Hydrodyanamic drag : Subsystem
  Product{4..7} (4 alike) : Product
  Scope2 : Scope
  Scope3 : Scope  NumInputPorts=4
  Scope5 : Scope
  Subsystem : Subsystem
  Sum : Sum
  Sum1 : Sum
  Translational Friction : fl_lib/Mechanical/Translational Elements/Translational Friction  brkwy_frc=25 N  brkwy_vel=0.1 m/s  Col_frc=20 N  visc_coef=100 N*s/m  v_specify=off  v_priority=None  v=0 m/s  v_nominal_specify=off  v_nominal_value=1  v_nominal_unit=m/s  f_specify=off  f_priority=None  f=0 N  f_nominal_specify=off  f_nominal_value=1  f_nominal_unit=N
      settings: InternalSimscapePortConfiguration="{\"Bottom\":[],\"Left\":[{\"id\":\"R\",\"label\":\"R\",\"type\":\"foundation.mechanical.translational.translational\"}],\"Right\":[{\"id\":\"C\",\"label\":\"C\",\"type\":\"foundation.mechanical.translational.translational\"}],\"Top\":[]}"
  quadratic force : Product
  quadratic moment : Product
  Out Bus Element : Outport  PortName=Drag  Element=Forces
  Out Bus Element1 : Outport  PortName=Drag  Element=Moments
  Out Bus Element2 : Outport  PortName=Drag  Element=LinearForce
  Out Bus Element3 : Outport  PortName=Drag  Element=LinearMoment
  wires:
  [oneminusWz] -> Product6/1, Product7/1
  Omega_b/1 -> Aerodynamic drag/2(Omega_b), Scope5/1, Hydrodyanamic drag/2(Omega_b), [wb]
  Velocity/1 -> Scope2/1, Hydrodyanamic drag/1(Velocity), Aerodynamic drag/1(Velocity), [Vb]
  Sum/1 -> quadratic force/2
  [Wz] -> Product4/1, Product5/1
  Hydrodyanamic drag/1(Force|_W) -> Product4/2  "hydro_f"
  quadratic force/1 -> Out Bus Element/1, Scope3/3
  Hydrodyanamic drag/2(Moment_W) -> Product5/2  "hydro_m"
  Aerodynamic drag/1(Force|_W) -> Product6/2  "aero_f"
  Aerodynamic drag/2(Moment_W) -> Product7/2  "Aero M"
  Subsystem/4(lambdaomega) -> quadratic moment/1
  Product6/1 -> Sum/2
  Altitude/1 -> Subsystem/1(Altitude)
  Product7/1 -> Sum1/2
  [Vb] -> Subsystem/2(v)
  Sum1/1 -> quadratic moment/2
  Product5/1 -> Sum1/1
  [wb] -> Subsystem/3(omega)
  Product4/1 -> Sum/1
  Subsystem/1(1mwz) -> [oneminusWz]
  Subsystem/2(W(z)) -> [Wz]
  Subsystem/3(lambdav) -> quadratic force/1
  quadratic moment/1 -> Out Bus Element1/1, Scope3/4
  Constant/1 -> Out Bus Element3/1, Out Bus Element2/1

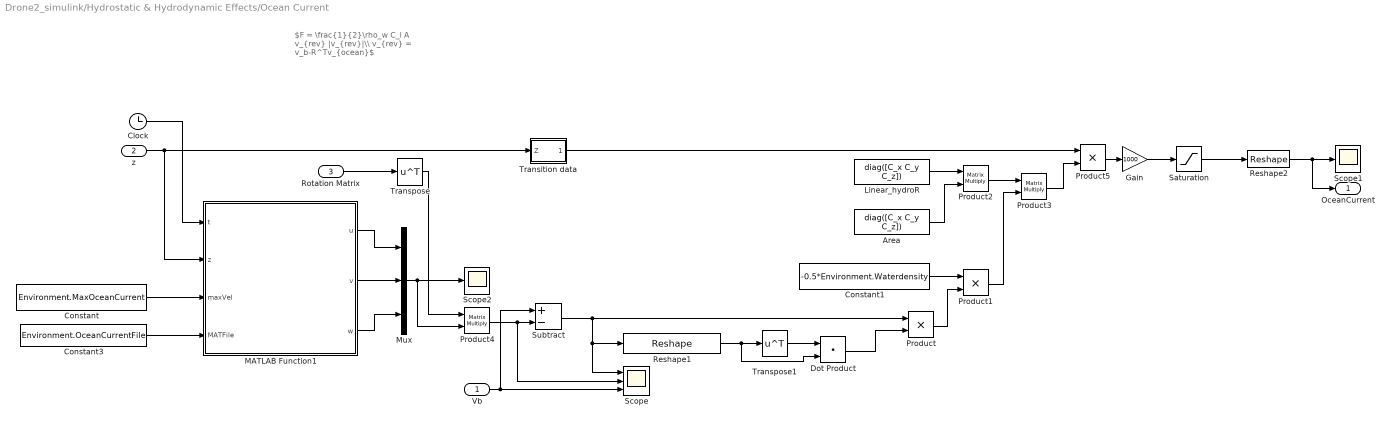
== system Drone2_simulink/Hydrostatic & Hydrodynamic Effects/Ocean Current ==
  note: $F = \frac{1}{2}\rho_w C_l A v_{rev} |v_{rev}|\\ v_{rev} = v_b-R^Tv_{ocean}$
  Vb : Inport
  z : Inport  Port=2
  Rotation Matrix : Inport  Port=3
  Area : Constant  Value=diag([C_x C_y C_z])  mask{C_x=Vehicle.Body.YZArea, C_y=Vehicle.Body.XZArea, C_z=Vehicle.Body.XYArea}
      mask prompts: C_x "Ax"; C_y "Ay"; C_z "Az"
      mask DialogControl DescGroupVar Prompt: Diagonal Matrix
      mask DialogControl DescTextVar Prompt: Provide values of diagonal element tp produce a diagonal matrix
      mask Display: disp('diag([Ax Ay Az])');
  Clock : Clock
  Constant : Constant  Value=Environment.MaxOceanCurrent
  Constant1 : Constant  Value=-0.5*Environment.Waterdensity
  Constant3 : Constant  Value=Environment.OceanCurrentFile  OutDataTypeStr=Bus: A
  Dot Product : DotProduct  OutDataTypeStr=Inherit: Inherit via internal rule
  Gain : Gain  Gain=1000
  Linear_hydroR : Constant  Value=diag([C_x C_y C_z])  mask{C_x=Environment.Ocean.cdx, C_y=Environment.Ocean.cdy, C_z=Environment.Ocean.cdz}
      mask prompts: C_x "Drag X"; C_y "Drag Y"; C_z "Drag Z"
      mask DialogControl DescGroupVar Prompt: Drag
      mask DialogControl DescTextVar Prompt: Provide values for linear or rotation drage to formulate a diagonal  drag matrix
      mask Display: disp('diag([C_x C_y C_z])');
  MATLAB Function1 : MATLAB Function  TreatAsAtomicUnit=on
  Mux : Mux  Inputs=3
  Product : Product
  Product1 : Product
  Product2 : Product  Multiplication=Matrix(*)
  Product3 : Product  Multiplication=Matrix(*)
  Product4 : Product  Multiplication=Matrix(*)
  Product5 : Product
  Reshape1 : Reshape  OutputDimensionality=Customize  OutputDimensions=[3,1]
  Reshape2 : Reshape  OutputDimensionality=Customize  OutputDimensions=[3,1]
  Saturation : Saturate  UpperLimit=5  LowerLimit=-5
  Scope : Scope  NumInputPorts=3
  Scope1 : Scope
  Scope2 : Scope
  Subtract : Sum  Inputs=+-
  Transition data : Subsystem
  Transpose : Math  Operator=transpose
  Transpose1 : Math  Operator=transpose
  OceanCurrent : Outport
  wires:
  Product4/1 -> Scope/2, Subtract/2
  MATLAB Function1/1(u) -> Mux/1
  Product2/1 -> Product3/1
  Constant3/1 -> MATLAB Function1/4(MATFile)
  Product/1 -> Product1/2
  Clock/1 -> MATLAB Function1/1(t)
  z/1 -> Transition data/1(Z), MATLAB Function1/2(z)
  MATLAB Function1/3(w) -> Mux/3
  Constant/1 -> MATLAB Function1/3(maxVel)
  Dot Product/1 -> Product/2
  MATLAB Function1/2(v) -> Mux/2
  Rotation Matrix/1 -> Transpose/1
  Transpose/1 -> Product4/1
  Mux/1 -> Product4/2, Scope2/1
  Vb/1 -> Scope/3, Subtract/1
  Transition data/1(W(z)) -> Product5/1
  Subtract/1 -> Reshape1/1, Scope/1, Product/1
  Linear_hydroR/1 -> Product2/1
  Reshape1/1 -> Transpose1/1, Dot Product/2
  Transpose1/1 -> Dot Product/1
  Area/1 -> Product2/2
  Product1/1 -> Product3/2
  Constant1/1 -> Product1/1
  Product3/1 -> Product5/2
  Product5/1 -> Gain/1
  Reshape2/1 -> Scope1/1, OceanCurrent/1
  Gain/1 -> Saturation/1
  Saturation/1 -> Reshape2/1

== system Drone2_simulink/Hydrostatic & Hydrodynamic Effects/Wind force ==
  note: $F = \frac{1}{2}\rho_w C_l A v_{rev} |v_{rev}|\\ v_{rev} = v_b-R^Tv_{ocean}$
  Vb : Inport
  z : Inport  Port=2
  Rotation Matrix : Inport  Port=3
  Area : Constant  Value=diag([C_x C_y C_z])  mask{C_x=Vehicle.Body.YZArea, C_y=Vehicle.Body.XZArea, C_z=Vehicle.Body.XYArea}
      mask prompts: C_x "Ax"; C_y "Ay"; C_z "Az"
      mask DialogControl DescGroupVar Prompt: Diagonal Matrix
      mask DialogControl DescTextVar Prompt: Provide values of diagonal element tp produce a diagonal matrix
      mask Display: disp('diag([Ax Ay Az])');
  Clock : Clock
  Constant : Constant  Value=Environment.Wind.mean
  Constant1 : Constant  Value=-0.5*Environment.Airdensity
  Constant2 : Constant
  Constant3 : Constant  Value=Environment.Wind.MAX
  Dot Product : DotProduct  OutDataTypeStr=Inherit: Inherit via internal rule
  Linear_AeroR : Constant  Value=diag([C_x C_y C_z])  mask{C_x=Environment.Wind.cdx, C_y=Environment.Wind.cdy, C_z=Environment.Wind.cdz}
      mask prompts: C_x "Drag X"; C_y "Drag Y"; C_z "Drag Z"
      mask DialogControl DescGroupVar Prompt: Drag
      mask DialogControl DescTextVar Prompt: Provide values for linear or rotation drage to formulate a diagonal  drag matrix
      mask Display: disp('diag([C_x C_y C_z])');
  Mux : Mux  Inputs=3
  Product : Product
  Product1 : Product
  Product2 : Product  Multiplication=Matrix(*)
  Product3 : Product  Multiplication=Matrix(*)
  Product4 : Product  Multiplication=Matrix(*)
  Product5 : Product
  Reshape1 : Reshape  OutputDimensionality=Customize  OutputDimensions=[3,1]
  Reshape2 : Reshape  OutputDimensionality=Customize  OutputDimensions=[3,1]
  Scope : Scope  NumInputPorts=3
  Scope1 : Scope
  Scope2 : Scope
  Subtract : Sum  Inputs=+-
  Subtract1 : Sum  Inputs=+-
  Transition data : Subsystem
  Transpose : Math  Operator=transpose
  Transpose1 : Math  Operator=transpose
  wind_disturbance : MATLAB Function  TreatAsAtomicUnit=on
  Wind Force : Outport
  wires:
  Rotation Matrix/1 -> Transpose/1
  Clock/1 -> wind_disturbance/1(t)
  Constant3/1 -> wind_disturbance/3(v_max)
  Constant/1 -> wind_disturbance/2(v_mean)
  Transpose/1 -> Product4/1
  Transition data/1(W(z)) -> Subtract1/2
  wind_disturbance/1(vx) -> Mux/1
  wind_disturbance/2(vy) -> Mux/2
  wind_disturbance/3(vz) -> Mux/3
  Mux/1 -> Scope2/1, Product4/2
  Vb/1 -> Scope/3, Subtract/1
  Product4/1 -> Scope/2, Subtract/2
  Subtract/1 -> Product/1, Scope/1, Reshape1/1
  Linear_AeroR/1 -> Product2/1
  Reshape1/1 -> Dot Product/2, Transpose1/1
  Transpose1/1 -> Dot Product/1
  Dot Product/1 -> Product/2
  Constant1/1 -> Product1/1
  Product/1 -> Product1/2
  Area/1 -> Product2/2
  Product1/1 -> Reshape2/1
  z/1 -> Transition data/1(Z)
  Constant2/1 -> Subtract1/1
  Product2/1 -> Product3/1
  Reshape2/1 -> Product3/2
  Product3/1 -> Product5/1
  Subtract1/1 -> Product5/2
  Product5/1 -> Scope1/1, Wind Force/1

== system Drone2_simulink/Physical_system/COB_data ==
  COBtranformation : sm_lib/Frames and Transforms/Rigid Transform  RotationMethod=None  FollAlignAxisA=+X  BaseAlignAxisA=+Y  FollAlignAxisB=+Y  BaseAlignAxisB=+Z  RotationStandardAxis=+Z  RotationAngle=0  RotationAngleUnits=deg  RotationArbitraryAxis=[0 0 1]  RotationSequenceAxes=FollowerAxes  RotationSequence=XYX  RotationSequenceAngles=[0 0 0]  RotationSequenceAnglesUnits=deg  RotationMatrix=[1 0 0;0 1 0;0 0 1]  Quaternion=[1 0 0 0]  TranslationMethod=Cartesian  TranslationCartesianOffset=[-0.00162 0.00068 0.005 ]  TranslationCartesianOffsetUnits=m  TranslationStandardAxis=+Z  TranslationStandardOffset=0  TranslationStandardOffsetUnits=m  TranslationROffset=0  TranslationROffsetUnits=m  TranslationThetaOffset=0  TranslationThetaOffsetUnits=deg  TranslationZOffset=0  TranslationZOffsetUnits=m
  COBtranformation1 : sm_lib/Frames and Transforms/Rigid Transform  Commented=on  RotationMethod=None  FollAlignAxisA=+X  BaseAlignAxisA=+Y  FollAlignAxisB=+Y  BaseAlignAxisB=+Z  RotationStandardAxis=+Z  RotationAngle=0  RotationAngleUnits=deg  RotationArbitraryAxis=[0 0 1]  RotationSequenceAxes=FollowerAxes  RotationSequence=XYX  RotationSequenceAngles=[0 0 0]  RotationSequenceAnglesUnits=deg  RotationMatrix=[1 0 0;0 1 0;0 0 1]  Quaternion=[1 0 0 0]  TranslationMethod=Cartesian  TranslationCartesianOffset=[-0.00192 0.00068 0.005 ]  TranslationCartesianOffsetUnits=m  TranslationStandardAxis=+Z  TranslationStandardOffset=0  TranslationStandardOffsetUnits=m  TranslationROffset=0  TranslationROffsetUnits=m  TranslationThetaOffset=0  TranslationThetaOffsetUnits=deg  TranslationZOffset=0  TranslationZOffsetUnits=m
  Coblocation : sm_lib/Body Elements/Graphic  GraphicType=Marker  MarkerShape=Sphere  MarkerSize=10  GraphicVisPropType=SimpleVisualProperties  GraphicDiffuseColor=[0 0 1]  GraphicOpacity=0.5  GraphicSpecularColor=[0.5 0.5 0.5 1.0]  GraphicAmbientColor=[0.15 0.15 0.15 1.0]  GraphicEmissiveColor=[0.0 0.0 0.0 1.0]  GraphicShininess=75
  Display : Display
  Display1 : Display
  Display2 : Display
  Inertia Sensor : sm_lib/Body Elements/Inertia Sensor  SensorExtent=BodyGroup  SpanWeldJoints=off  ExcludeGroundedBodies=off  MeasurementFrame=Attached  SenseMass=on  SenseCenterOfMass=on  SenseInertiaMatrix=on  SenseCenteredInertiaMatrix=off  SensePrincipalInertiaMatrix=off  SenseRotationMatrix=off  GraphicType=PrincipalInertiaFrame  PrincipalInertiaFrameSize=20  GraphicVisPropType=SimpleVisualProperties  GraphicDiffuseColor=[0.5 0.5 0.5]  GraphicOpacity=1  GraphicSpecularColor=[0.5 0.5 0.5 1.0]  GraphicAmbientColor=[0.15 0.15 0.15 1.0]  GraphicEmissiveColor=[0.0 0.0 0.0 1.0]  GraphicShininess=75
  PS-Simulink Converter : nesl_utility/PS-Simulink Converter  PhysicalDomain=network_engine_domain  SubClassName=ps_output  LeftPortType=input  RightPortType=output  PseudoPeriodic=off  Frequencies=[]  VectorFormat=inherit  Unit=inherit  AffineConversion=off
  PS-Simulink Converter1 : nesl_utility/PS-Simulink Converter  PhysicalDomain=network_engine_domain  SubClassName=ps_output  LeftPortType=input  RightPortType=output  PseudoPeriodic=off  Frequencies=[]  VectorFormat=inherit  Unit=inherit  AffineConversion=off
  PS-Simulink Converter2 : nesl_utility/PS-Simulink Converter  PhysicalDomain=network_engine_domain  SubClassName=ps_output  LeftPortType=input  RightPortType=output  PseudoPeriodic=off  Frequencies=[]  VectorFormat=inherit  Unit=inherit  AffineConversion=off
  COB : PMIOPort  Side=Left
  Base : PMIOPort  Port=2  Side=Left
  wires:
  PS-Simulink Converter/1 -> Display/1
  PS-Simulink Converter1/1 -> Display1/1
  PS-Simulink Converter2/1 -> Display2/1
  connections:
  COB/RConn1 -- Inertia Sensor/LConn1 -- COBtranformation/RConn1 -- Coblocation/RConn1
  Base/RConn1 -- COBtranformation/LConn1
  PS-Simulink Converter/LConn1 -- Inertia Sensor/RConn1
  PS-Simulink Converter1/LConn1 -- Inertia Sensor/RConn2
  PS-Simulink Converter2/LConn1 -- Inertia Sensor/RConn3

== system Drone2_simulink/Physical_system/COM_Data ==
  " CoM Measurements" : Subsystem
      settings: PortSchema="{\"entries\":[{\"content\":{\"sides\":[{\"content\":{\"connectorIds\":[]},\"type\":\"ConnectorPlacement.EquallySpacedRectSide\",\"uuid\":\"41b17865-a6b4-4c1a-ad12-0699c57309aa\"},{\"content\":{\"connectorIds\":[\"Out1\",\"Out2\"],\"side\":\"RIGHT\"},\"type\":\"ConnectorPlacement.EquallySpacedRectSide\",\"uuid\":\"edfedad4-b08a-45ae-9215-ce29af402ac0\"},{\"content\":{\"connectorIds\":[\"LConn1\"],\"side\":\"TOP\"},\"type\":\"ConnectorPlacement.EquallySpacedRectSide\",\"uuid\":\"e431dbfc-8157-4a96-9a26-4b41afc24a27\"}]},\"type\":\"ConnectorPlacement.EquallySpacedConnector\",\"uuid\":\"fb33b9ce-c03b-4394-a7d9-78d177de3027\"}],\"packageUris\":[\"http://schema.mathworks.com/mf0/Connector/19700101\"],\"version\":\"1.0\"}"
  COMtransformation : sm_lib/Frames and Transforms/Rigid Transform  RotationMethod=None  FollAlignAxisA=+X  BaseAlignAxisA=+Y  FollAlignAxisB=+Y  BaseAlignAxisB=+Z  RotationStandardAxis=+Z  RotationAngle=0  RotationAngleUnits=deg  RotationArbitraryAxis=[0 0 1]  RotationSequenceAxes=FollowerAxes  RotationSequence=XYX  RotationSequenceAngles=[0 0 0]  RotationSequenceAnglesUnits=deg  RotationMatrix=[1 0 0;0 1 0;0 0 1]  Quaternion=[1 0 0 0]  TranslationMethod=Cartesian  TranslationCartesianOffset="[-0.003  0.00068 -0.00442]"  TranslationCartesianOffsetUnits=m  TranslationStandardAxis=+Z  TranslationStandardOffset=0  TranslationStandardOffsetUnits=m  TranslationROffset=0  TranslationROffsetUnits=m  TranslationThetaOffset=0  TranslationThetaOffsetUnits=deg  TranslationZOffset=0  TranslationZOffsetUnits=m
  Derived Measurements : Subsystem
  Graphic : sm_lib/Body Elements/Graphic  GraphicType=Marker  MarkerShape=Sphere  MarkerSize=10  GraphicVisPropType=SimpleVisualProperties  GraphicDiffuseColor=[1 0 0]  GraphicOpacity=1  GraphicSpecularColor=[0.5 0.5 0.5 1.0]  GraphicAmbientColor=[0.15 0.15 0.15 1.0]  GraphicEmissiveColor=[0.0 0.0 0.0 1.0]  GraphicShininess=75
  CoM : PMIOPort  Side=Left
  Base : PMIOPort  Port=2  Side=Right
  Out Bus Element : Outport  PortName=COM  Element=Body
  Out Bus Element1 : Outport  PortName=COM  Element=Derived
  Out Bus Element2 : Outport  PortName=COM  Element=World
  wires:
  " CoM Measurements"/2(World) -> Derived Measurements/2(World), Out Bus Element2/1
  " CoM Measurements"/1(Body) -> Derived Measurements/1(Body), Out Bus Element/1
  Derived Measurements/1(Derived) -> Out Bus Element1/1
  connections:
  CoM/RConn1 -- Graphic/RConn1 -- " CoM Measurements"/LConn1 -- COMtransformation/RConn1
  COMtransformation/LConn1 -- Base/RConn1

== system Drone2_simulink/Physical_system/Drone_Assembly ==
  In Bus Element : Inport  PortName=Actuator  Element=Aerial
  In Bus Element1 : Inport  PortName=Actuator  Element=Underwater
  In Bus Element2 : Inport  PortName=Actuator  Element=BuoyancyForce
  Arm Assembly : Subsystem
  Cylinder_Assembly : Subsystem
      mask Display: image('Cylinder_Assembly.PNG');
  Scope : Scope
  Scope1 : Scope
  Scope2 : Scope
  ThrusterAssembly : Subsystem  mask{Stiffness=Vehicle.Thruster.Stiffness, Damping=Vehicle.Thruster.Damping, Gl=CCW, Gr=CW, MaxThrust=Vehicle.Thruster.MaxForwardThrust, MinThrust=Vehicle.Thruster.MaxReverseThrust, MaxTorque=Vehicle.Thruster.Maxtorque, MinTorque=0}
      mask prompts: Gl "Thruster L rot"; Gr "Thruster R rot"
      mask DialogControl Container4 Prompt: Thruster Data
      mask DialogControl Container5 Prompt: Thrust force
      mask DialogControl Container6 Prompt: Torque
      mask Display: image('T200-THRUSTER-housing.JPG');
  FromCO : PMIOPort  Side=Left
  Hull : PMIOPort  Port=2  Side=Left
  buoyancy : Outport
  wires:
  Cylinder_Assembly/1(Buoyancy) -> buoyancy/1
  In Bus Element/1 -> Scope1/1, Arm Assembly/1(Aerial)
  In Bus Element1/1 -> Scope2/1, ThrusterAssembly/1(Actuator)
  In Bus Element2/1 -> Scope/1, Cylinder_Assembly/1(Force)
  connections:
  FromCO/RConn1 -- Arm Assembly/RConn1 -- ThrusterAssembly/LConn1 -- Cylinder_Assembly/LConn1
  Hull/RConn1 -- Cylinder_Assembly/LConn2
